simulink model "EngineController"  (Simulink 7.7)
settings: Solver=ode45  StartTime=0.0  StopTime=10.0  RelTol=1e-3
settings Model: Creator=META-DEMO  LastModifiedBy=jscott

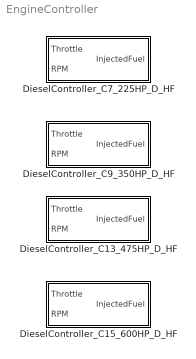
== system EngineController ==
  DieselController_C13_475HP_D_HF : Subsystem
  DieselController_C15_600HP_D_HF : Subsystem
  DieselController_C7_225HP_D_HF : Subsystem
  DieselController_C9_350HP_D_HF : Subsystem

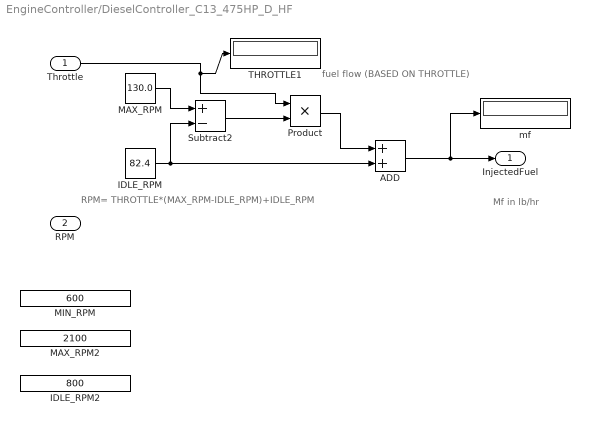
== system EngineController/DieselController_C13_475HP_D_HF ==
  note: Mf in lb/hr
  note: fuel flow
      | (BASED ON THROTTLE)
  note: RPM= THROTTLE*(MAX_RPM-IDLE_RPM)+IDLE_RPM
  Throttle : Inport
  RPM : Inport  Port=2
  ADD : Sum
  IDLE_RPM : Constant  Value=82.4
  IDLE_RPM2 : Constant  Value=800
  MAX_RPM : Constant  Value=130.0
  MAX_RPM2 : Constant  Value=2100
  MIN_RPM : Constant  Value=600
  Product : Product  RndMeth=Zero
  Subtract2 : Sum  Inputs=+-
  THROTTLE1 : Display
  mf : Display
  InjectedFuel : Outport
  wires:
  MAX_RPM/1 -> Subtract2/1
  IDLE_RPM/1 -> Subtract2/2, ADD/2
  Throttle/1 -> Product/1, THROTTLE1/1
  Subtract2/1 -> Product/2
  Product/1 -> ADD/1
  ADD/1 -> InjectedFuel/1, mf/1

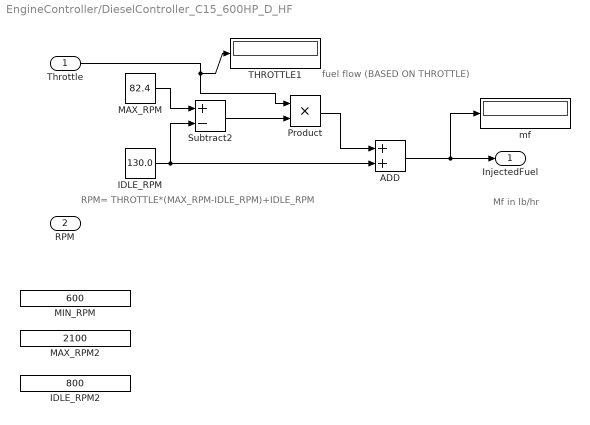
== system EngineController/DieselController_C15_600HP_D_HF ==
  note: Mf in lb/hr
  note: fuel flow
      | (BASED ON THROTTLE)
  note: RPM= THROTTLE*(MAX_RPM-IDLE_RPM)+IDLE_RPM
  Throttle : Inport
  RPM : Inport  Port=2
  ADD : Sum
  IDLE_RPM : Constant  Value=130.0
  IDLE_RPM2 : Constant  Value=800
  MAX_RPM : Constant  Value=82.4
  MAX_RPM2 : Constant  Value=2100
  MIN_RPM : Constant  Value=600
  Product : Product  RndMeth=Zero
  Subtract2 : Sum  Inputs=+-
  THROTTLE1 : Display
  mf : Display
  InjectedFuel : Outport
  wires:
  MAX_RPM/1 -> Subtract2/1
  IDLE_RPM/1 -> Subtract2/2, ADD/2
  Throttle/1 -> Product/1, THROTTLE1/1
  Subtract2/1 -> Product/2
  Product/1 -> ADD/1
  ADD/1 -> InjectedFuel/1, mf/1

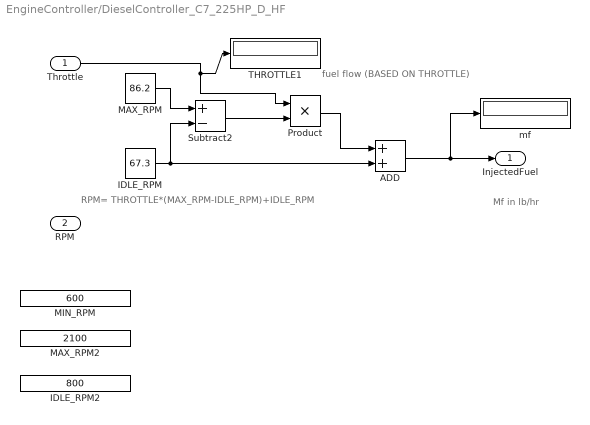
== system EngineController/DieselController_C7_225HP_D_HF ==
  note: Mf in lb/hr
  note: fuel flow
      | (BASED ON THROTTLE)
  note: RPM= THROTTLE*(MAX_RPM-IDLE_RPM)+IDLE_RPM
  Throttle : Inport
  RPM : Inport  Port=2
  ADD : Sum
  IDLE_RPM : Constant  Value=67.3
  IDLE_RPM2 : Constant  Value=800
  MAX_RPM : Constant  Value=86.2
  MAX_RPM2 : Constant  Value=2100
  MIN_RPM : Constant  Value=600
  Product : Product  RndMeth=Zero
  Subtract2 : Sum  Inputs=+-
  THROTTLE1 : Display
  mf : Display
  InjectedFuel : Outport
  wires:
  MAX_RPM/1 -> Subtract2/1
  IDLE_RPM/1 -> Subtract2/2, ADD/2
  Throttle/1 -> Product/1, THROTTLE1/1
  Subtract2/1 -> Product/2
  Product/1 -> ADD/1
  ADD/1 -> InjectedFuel/1, mf/1

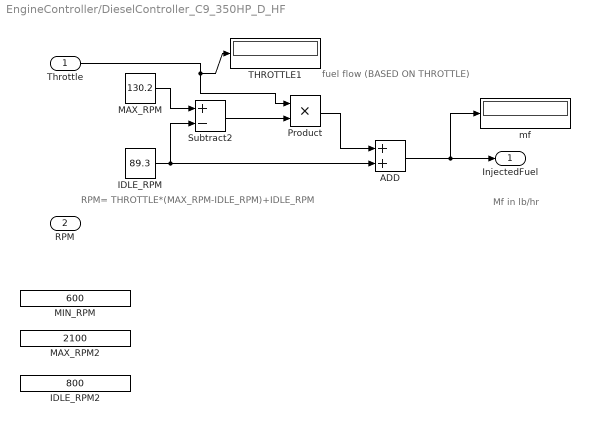
== system EngineController/DieselController_C9_350HP_D_HF ==
  note: Mf in lb/hr
  note: fuel flow
      | (BASED ON THROTTLE)
  note: RPM= THROTTLE*(MAX_RPM-IDLE_RPM)+IDLE_RPM
  Throttle : Inport
  RPM : Inport  Port=2
  ADD : Sum
  IDLE_RPM : Constant  Value=89.3
  IDLE_RPM2 : Constant  Value=800
  MAX_RPM : Constant  Value=130.2
  MAX_RPM2 : Constant  Value=2100
  MIN_RPM : Constant  Value=600
  Product : Product  RndMeth=Zero
  Subtract2 : Sum  Inputs=+-
  THROTTLE1 : Display
  mf : Display
  InjectedFuel : Outport
  wires:
  MAX_RPM/1 -> Subtract2/1
  IDLE_RPM/1 -> Subtract2/2, ADD/2
  Throttle/1 -> Product/1, THROTTLE1/1
  Subtract2/1 -> Product/2
  Product/1 -> ADD/1
  ADD/1 -> InjectedFuel/1, mf/1
